simulink subsystem "DCM"  (R2024b)
settings: Solver=VariableStepAuto  StartTime=0.0  StopTime=10.0  RelTol=1e-3
undefined symbols (not defined in the file or in its folder): dcm
settings Model: Creator=matth  LastModifiedBy=matth

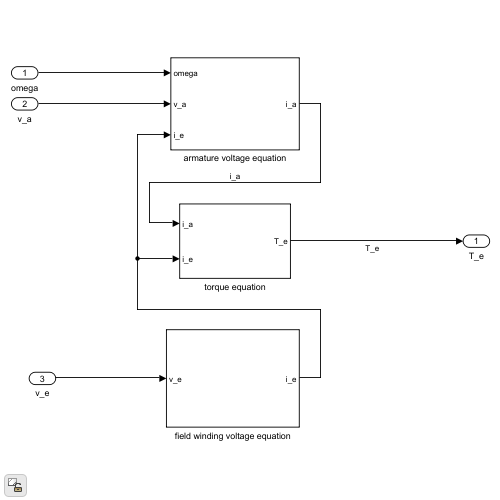
[thumbnail: Simulink's stored preview of the top-level diagram]
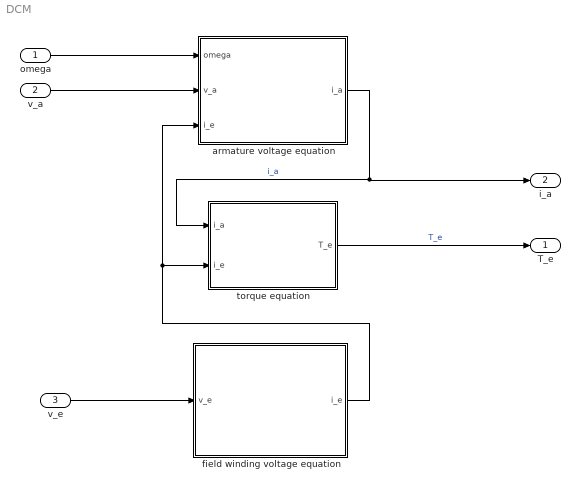
== system DCM ==
  omega : Inport
  v_a : Inport  Port=2
  v_e : Inport  Port=3
  armature voltage equation : Subsystem
  field winding voltage equation : Subsystem
  torque equation : Subsystem
  T_e : Outport
  i_a : Outport  Port=2
  wires:
  omega/1 -> armature voltage equation/1(omega)
  v_a/1 -> armature voltage equation/2(v_a)
  armature voltage equation/1(i_a) -> torque equation/1(i_a), i_a/1  "i_a"
  field winding voltage equation/1(i_e) -> armature voltage equation/3(i_e), torque equation/2(i_e)
  v_e/1 -> field winding voltage equation/1(v_e)
  torque equation/1(T_e) -> T_e/1  "T_e"

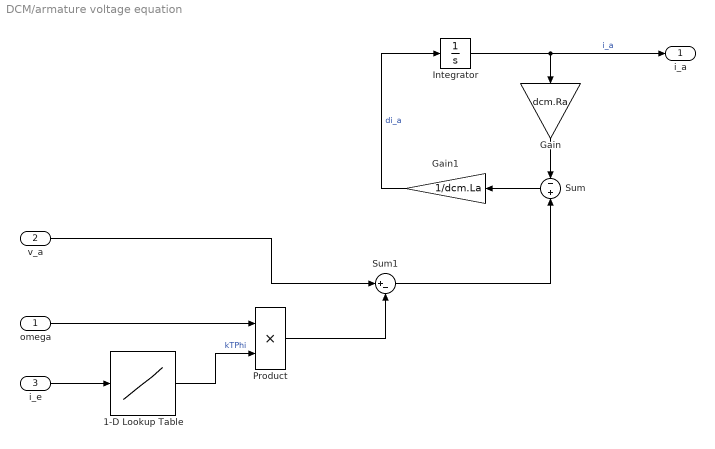
== system DCM/armature voltage equation ==
  omega : Inport
  v_a : Inport  Port=2
  i_e : Inport  Port=3
  1-D Lookup Table : Lookup_n-D  NumberOfTableDimensions=1  BreakpointsForDimension1=dcm.if_tab  Table=dcm.KPhi_tab  InternalRulePriority=Speed  RndMeth=Simplest
  Gain : Gain  Gain=dcm.Ra
  Gain1 : Gain  Gain=1/dcm.La
  Integrator : Integrator  InitialCondition=dcm.ia0
  Product : Product
  Sum : Sum  Inputs=-|+
  Sum1 : Sum  Inputs=|+-
  i_a : Outport
  wires:
  Gain/1 -> Sum/1
  Integrator/1 -> Gain/1, i_a/1  "i_a"
  omega/1 -> Product/1
  Sum1/1 -> Sum/2
  Gain1/1 -> Integrator/1  "di_a"
  Product/1 -> Sum1/2
  Sum/1 -> Gain1/1
  v_a/1 -> Sum1/1
  1-D Lookup Table/1 -> Product/2  "kTPhi"
  i_e/1 -> 1-D Lookup Table/1

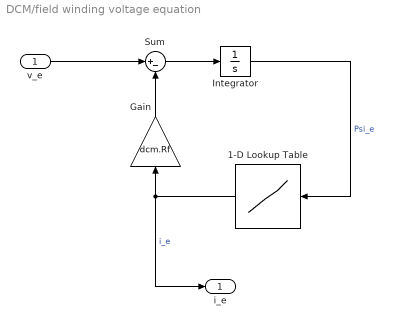
== system DCM/field winding voltage equation ==
  v_e : Inport
  1-D Lookup Table : Lookup_n-D  NumberOfTableDimensions=1  BreakpointsForDimension1=dcm.psiftab  Table=dcm.iftab  InternalRulePriority=Speed  RndMeth=Simplest
  Gain : Gain  Gain=dcm.Rf
  Integrator : Integrator  InitialCondition=dcm.psie0
  Sum : Sum  Inputs=|+-
  i_e : Outport
  wires:
  Integrator/1 -> 1-D Lookup Table/1  "Psi_e"
  v_e/1 -> Sum/1
  1-D Lookup Table/1 -> Gain/1, i_e/1  "i_e"
  Sum/1 -> Integrator/1
  Gain/1 -> Sum/2

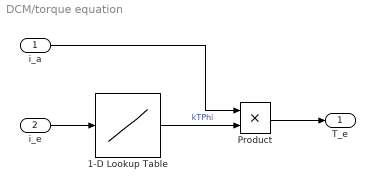
== system DCM/torque equation ==
  i_a : Inport
  i_e : Inport  Port=2
  1-D Lookup Table : Lookup_n-D  NumberOfTableDimensions=1  BreakpointsForDimension1=dcm.if_tab  Table=dcm.KPhi_tab  InternalRulePriority=Speed  RndMeth=Simplest
  Product : Product
  T_e : Outport
  wires:
  i_a/1 -> Product/1
  Product/1 -> T_e/1
  i_e/1 -> 1-D Lookup Table/1
  1-D Lookup Table/1 -> Product/2  "kTPhi"
